simulink model "PVWIND"  (R2018a)
settings: Solver=FixedStepAuto  StartTime=0.0  StopTime=8  FixedStep=1e-4  RelTol=1e-3  EnableMultiTasking=on
InitFcn:
  | %clear all ;
  | %clc;
  | 
  | %%Wind System%%
  | 
  | %wind speed
  | Z_data=10;
  | Z_hub=85;
  | Z_0=0.03;
  | 
  | %Turbine
  | R_=45;
  | G=100;
  | lambda_opt=7.07;
  | Rho=1.225;
  | J=254;
  | f=0.01;
  | 
  | %RL filter;
  | 
  | fs=10000;
  | fe=50;
  | Ws=2*pi*fe;
  | Pres=3e6;
  | L=0.75e-3;
  | R=0.075;
  | c=38e-3;
  | 
  | %Commande CCR;
  | 
  | Id_=0;
  | Vdc_=1200;
  | %Vq_=0;
  | tr=0.001;
  | kp=3*L/tr;
  | ki=3*R/tr;
  | 
  | %CCM Commande;
  | 
  | p=2;
  | Tr=0.02;
  | Lfs=121e-6;
  | Lfr=57.3e-6;
  | Lm=12.12e-3;
  | m=1;
  | Ls=Lfs+Lm;
  | Lr=Lfr+m*Lm;
  | sigma=1-(m*Lm)^2/(Ls*Lr);
  | Rr=3.82e-3;
  | Rs=2.97e-3;
  | kpr=3*sigma*Lr/Tr;
  | kir=3*Rr/Tr;
  | Qs_ref=0;
  | 
  | %%PV SYSTEM%%
  | 
  | % T_cellule;
  | NOCT=45;
  | 
  | %PV module;
  | Ki=5e-4;
  | q=1.6e-19;
  | K=1.38e-23;
  | n=1.3;
  | Eg0=1.12;
  | Rs=.1;
  | Rp=515;
  | Tn=298.15;
  | Gn=1000;
  | Voc=46.5;
  | Isc=9.68;
  | Ns=72;
  | 
  | % Boost converter;
  | dv=3.1;   %53.85;
  | di=0.16;  %0.2053;
  | F=10000;
  | T=1/F;
  | %Vs=398;
  | Vab=690;         %sqrt(3)*Vs;
  | Vdc=1200;       %2*sqrt(2)*Vab/sqrt(3);
  | Vpv=303.2;
  | a=1-Vpv/Vdc;
  | Pn=350*40;
  | r=Vdc*Vdc/Pn;
  | l=0.5*Vpv*a*T/di;              %80e-3;
  | C=0.5*Vdc*a*T/(dv*r);       % 10e-6;
  | 
  | 
  | %Control PWM
  | Vgq=690/sqrt(3);
  | Fs=5000;
  | Ig=2*Pn/(3*690/sqrt(3)*sqrt(2));
  | dIg=0.05*Ig;
  | L1=690/(6*sqrt(2)*Fs*dIg);
  | R1=0.01;
  | 
  | 
  | tr1=1e-5;
  | Tau=tr1/3;
  | ki1=R1/Tau/Vgq;
  | kp1=L1/Tau/Vgq;
undefined symbols (not defined in the file or in its folder): sigbuilder_block
libraries: simulink x10, powerlib_meascontrol x10
(part 1 of 2)
settings Model: Creator=PC  LastModifiedBy=yassine
settings DataIOCC: SaveFormat=Array
settings OptimizationCC: LifeSpan=inf
settings DebuggingCC: SFUnexpectedBacktrackingDiag=warning  SFNoUnconditionalDefaultTransitionDiag=warning
settings CodeAppCC: StateflowObjectComments=on
settings GRTTargetCC: TargetLangStandard=C89/C90 (ANSI)
settings ConfigComp: CovMetricSettings=dw  CovSaveCumulativeToWorkspaceVar=on  CovSaveSingleToWorkspaceVar=on  CovExternalEMLEnable=off

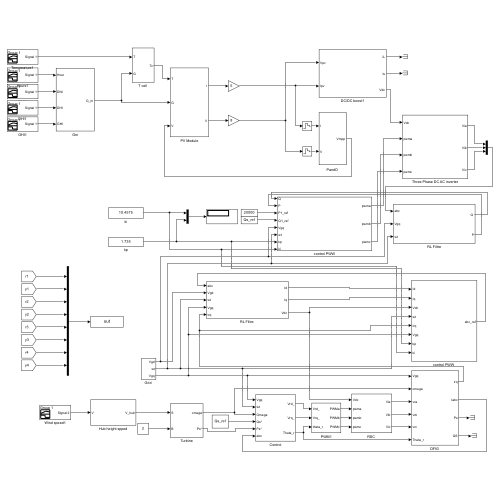
[thumbnail: Simulink's stored preview of the top-level diagram]
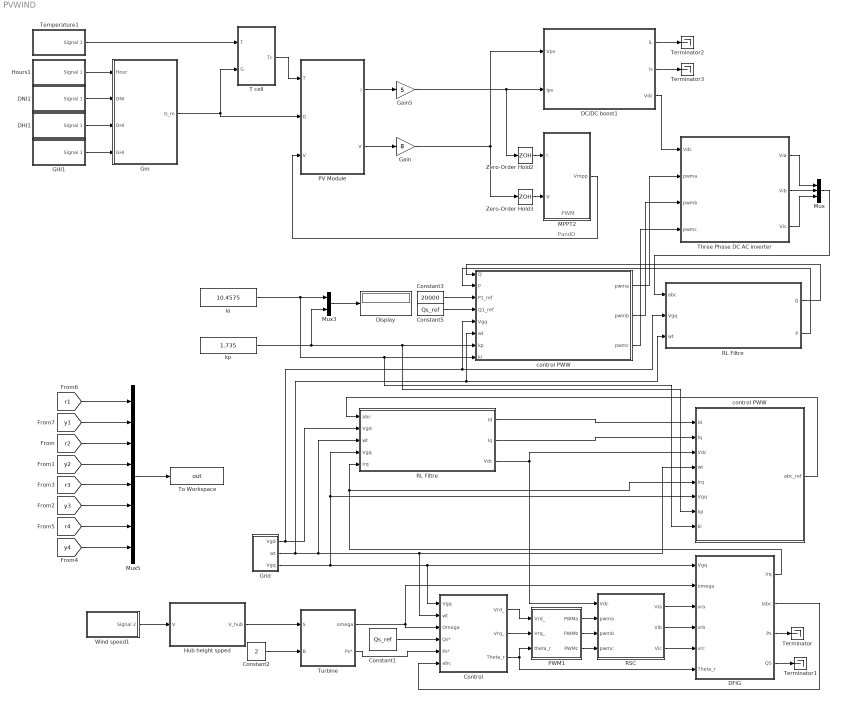
== system PVWIND ==
  note: PWM
  note: PandO
  Constant1 : Constant  Value=Qs_ref
  Constant2 : Constant  Value=2
  Constant3 : Constant  Value=20000
  Constant5 : Constant  Value=Qs_ref
  Control : Subsystem
  DC/DC boost1 : Subsystem
  "DFIG " : Subsystem
  DHI1 : Subsystem  Tag=STV Subsys  LoadFcn=sigbuilder_block('load');  StartFcn=sigbuilder_block('start');  StopFcn=sigbuilder_block('stop');  ClipboardFcn=sigbuilder_block('clipboard');  mask(Sigbuilder block){tuvar=[0:10]}
      mask help: Simulink:masks:SigbuilderBlock_MD
      mask init:
      | if ~strcmp(get_param(bdroot(gcbh),'SimulationStatus'),'stopped') tuvar = sigbuilder_block('maskInit'); end
      settings: CopyFcn=sigbuilder_block('copy');  DeleteFcn=sigbuilder_block('delete');  ModelCloseFcn=sigbuilder_block('modelClose');  PreSaveFcn=sigbuilder_block('preSave');  PauseFcn=sigbuilder_block('pause');  ContinueFcn=sigbuilder_block('continue');  NameChangeFcn=sigbuilder_block('namechange');  OpenFcn=sigbuilder_block('open',[303.6 90.6 550.8 400.2 ]);  CloseFcn=sigbuilder_block('close');
      mask Display: plot(0, 0, 100, 100,[2, 2, 32, 32, 2], [68, 8, 8, 68, 68],[32, 2], [38, 38], [32, 19, 2],[53, 60, 44], [32, 17, 17, 2],[16, 16, 31, 31]);txt = getActiveGroup(gcbh);text(2, 100, txt,'verticalAlignment', 'top');
  DNI1 : Subsystem  Tag=STV Subsys  LoadFcn=sigbuilder_block('load');  StartFcn=sigbuilder_block('start');  StopFcn=sigbuilder_block('stop');  ClipboardFcn=sigbuilder_block('clipboard');  mask(Sigbuilder block){tuvar=[0:10]}
      mask help: Simulink:masks:SigbuilderBlock_MD
      mask init:
      | if ~strcmp(get_param(bdroot(gcbh),'SimulationStatus'),'stopped') tuvar = sigbuilder_block('maskInit'); end
      settings: CopyFcn=sigbuilder_block('copy');  DeleteFcn=sigbuilder_block('delete');  ModelCloseFcn=sigbuilder_block('modelClose');  PreSaveFcn=sigbuilder_block('preSave');  PauseFcn=sigbuilder_block('pause');  ContinueFcn=sigbuilder_block('continue');  NameChangeFcn=sigbuilder_block('namechange');  OpenFcn=sigbuilder_block('open',[446.4 127.8 550.8 400.2 ]);  CloseFcn=sigbuilder_block('close');
      mask Display: plot(0, 0, 100, 100,[2, 2, 32, 32, 2], [68, 8, 8, 68, 68],[32, 2], [38, 38], [32, 19, 2],[53, 60, 44], [32, 17, 17, 2],[16, 16, 31, 31]);txt = getActiveGroup(gcbh);text(2, 100, txt,'verticalAlignment', 'top');
  Display : Display
  GHI1 : Subsystem  Tag=STV Subsys  LoadFcn=sigbuilder_block('load');  StartFcn=sigbuilder_block('start');  StopFcn=sigbuilder_block('stop');  ClipboardFcn=sigbuilder_block('clipboard');  mask(Sigbuilder block){tuvar=[0:10]}
      mask help: Simulink:masks:SigbuilderBlock_MD
      mask init:
      | if ~strcmp(get_param(bdroot(gcbh),'SimulationStatus'),'stopped') tuvar = sigbuilder_block('maskInit'); end
      settings: CopyFcn=sigbuilder_block('copy');  DeleteFcn=sigbuilder_block('delete');  ModelCloseFcn=sigbuilder_block('modelClose');  PreSaveFcn=sigbuilder_block('preSave');  PauseFcn=sigbuilder_block('pause');  ContinueFcn=sigbuilder_block('continue');  NameChangeFcn=sigbuilder_block('namechange');  OpenFcn=sigbuilder_block('open',[431.4 162.6 550.8 400.2 ]);  CloseFcn=sigbuilder_block('close');
      mask Display: plot(0, 0, 100, 100,[2, 2, 32, 32, 2], [68, 8, 8, 68, 68],[32, 2], [38, 38], [32, 19, 2],[53, 60, 44], [32, 17, 17, 2],[16, 16, 31, 31]);txt = getActiveGroup(gcbh);text(2, 100, txt,'verticalAlignment', 'top');
  Gain : Gain  Gain=8
  Gain5 : Gain  Gain=5
  Gm : Subsystem
  "Grid " : Subsystem
  Hours1 : Subsystem  Tag=STV Subsys  LoadFcn=sigbuilder_block('load');  StartFcn=sigbuilder_block('start');  StopFcn=sigbuilder_block('stop');  ClipboardFcn=sigbuilder_block('clipboard');  mask(Sigbuilder block){tuvar=[0:10]}
      mask help: Simulink:masks:SigbuilderBlock_MD
      mask init:
      | if ~strcmp(get_param(bdroot(gcbh),'SimulationStatus'),'stopped') tuvar = sigbuilder_block('maskInit'); end
      settings: CopyFcn=sigbuilder_block('copy');  DeleteFcn=sigbuilder_block('delete');  ModelCloseFcn=sigbuilder_block('modelClose');  PreSaveFcn=sigbuilder_block('preSave');  PauseFcn=sigbuilder_block('pause');  ContinueFcn=sigbuilder_block('continue');  NameChangeFcn=sigbuilder_block('namechange');  OpenFcn=sigbuilder_block('open',[446.4 139.2 550.8 400.2 ]);  CloseFcn=sigbuilder_block('close');
      mask Display: plot(0, 0, 100, 100,[2, 2, 32, 32, 2], [68, 8, 8, 68, 68],[32, 2], [38, 38], [32, 19, 2],[53, 60, 44], [32, 17, 17, 2],[16, 16, 31, 31]);txt = getActiveGroup(gcbh);text(2, 100, txt,'verticalAlignment', 'top');
  Hub height spped : Subsystem
  MPPT2 : Subsystem
  Mux : Mux  Inputs=3
  Mux3 : Mux  Inputs=2
  Mux5 : Mux  Inputs=8
  PV Module : Subsystem
  PWM1 : Subsystem
  RL Filtre : Subsystem
  "RL Filtre " : Subsystem
  "RSC " : Subsystem
  "T cell " : Subsystem
  Temperature1 : Subsystem  Tag=STV Subsys  LoadFcn=sigbuilder_block('load');  StartFcn=sigbuilder_block('start');  StopFcn=sigbuilder_block('stop');  ClipboardFcn=sigbuilder_block('clipboard');  mask(Sigbuilder block){tuvar=[0:10]}
      mask help: Simulink:masks:SigbuilderBlock_MD
      mask init:
      | if ~strcmp(get_param(bdroot(gcbh),'SimulationStatus'),'stopped') tuvar = sigbuilder_block('maskInit'); end
      settings: CopyFcn=sigbuilder_block('copy');  DeleteFcn=sigbuilder_block('delete');  ModelCloseFcn=sigbuilder_block('modelClose');  PreSaveFcn=sigbuilder_block('preSave');  PauseFcn=sigbuilder_block('pause');  ContinueFcn=sigbuilder_block('continue');  NameChangeFcn=sigbuilder_block('namechange');  OpenFcn=sigbuilder_block('open',[492.6 104.4 550.8 400.2 ]);  CloseFcn=sigbuilder_block('close');
      mask Display: plot(0, 0, 100, 100,[2, 2, 32, 32, 2], [68, 8, 8, 68, 68],[32, 2], [38, 38], [32, 19, 2],[53, 60, 44], [32, 17, 17, 2],[16, 16, 31, 31]);txt = getActiveGroup(gcbh);text(2, 100, txt,'verticalAlignment', 'top');
  Terminator{,1..3} (4 alike) : Terminator
  Three Phase DC AC inverter : Subsystem
  To Workspace : ToWorkspace  VariableName=out  SaveFormat=Timeseries  SampleTime=-1
  Turbine : Subsystem
  Wind speed1 : Subsystem  Tag=STV Subsys  LoadFcn=sigbuilder_block('load');  StartFcn=sigbuilder_block('start');  StopFcn=sigbuilder_block('stop');  ClipboardFcn=sigbuilder_block('clipboard');  mask(Sigbuilder block){tuvar=[0:10]}
      mask help: Simulink:masks:SigbuilderBlock_MD
      mask init:
      | if ~strcmp(get_param(bdroot(gcbh),'SimulationStatus'),'stopped') tuvar = sigbuilder_block('maskInit'); end
      settings: CopyFcn=sigbuilder_block('copy');  DeleteFcn=sigbuilder_block('delete');  ModelCloseFcn=sigbuilder_block('modelClose');  PreSaveFcn=sigbuilder_block('preSave');  PauseFcn=sigbuilder_block('pause');  ContinueFcn=sigbuilder_block('continue');  NameChangeFcn=sigbuilder_block('namechange');  OpenFcn=sigbuilder_block('open',[363 165 550.8 400.2 ]);  CloseFcn=sigbuilder_block('close');
      mask Display: plot(0, 0, 100, 100,[2, 2, 32, 32, 2], [68, 8, 8, 68, 68],[32, 2], [38, 38], [32, 19, 2],[53, 60, 44], [32, 17, 17, 2],[16, 16, 31, 31]);txt = getActiveGroup(gcbh);text(2, 100, txt,'verticalAlignment', 'top');
  Zero-Order Hold2 : ZeroOrderHold  SampleTime=1e-4
  Zero-Order Hold3 : ZeroOrderHold  SampleTime=1e-4
  control PWW : Subsystem
  "control PWW " : Subsystem
  ki : Constant  Value=10.4575
  kp : Constant  Value=1.735
  wires:
  "RSC "/1(Via) -> "DFIG "/3(vra)
  "RSC "/2(Vib) -> "DFIG "/4(vrb)
  "RSC "/3(Vic) -> "DFIG "/5(vrc)
  "RL Filtre "/3(Vdc) -> "RSC "/1(Vdc), "control PWW "/3(Vdc)
  PWM1/2(PWMb) -> "RSC "/3(pwmb)
  Control/1(Vrd_) -> PWM1/1(Vrd_)
  Control/2(Vrq_) -> PWM1/2(Vrq_)
  PWM1/1(PWMa) -> "RSC "/2(pwma)
  PWM1/3(PWMc) -> "RSC "/4(pwmc)
  "Grid "/3(Vgq) -> Control/1(Vgq), "DFIG "/1(Vgq), "RL Filtre "/4(Vgq), "control PWW "/6(Vgq)
  Control/3(Theta_r) -> "DFIG "/6(Theta_r), PWM1/3(theta_r)
  "DFIG "/2(Iabc) -> Control/6(abc)
  Turbine/1(omega) -> "DFIG "/2(omega), Control/3(Omega)
  "control PWW "/1(abc_ref) -> "RL Filtre "/1(abc)
  "RL Filtre "/1(Id) -> "control PWW "/1(Id)
  "RL Filtre "/2(Iq) -> "control PWW "/2(Iq)
  "DFIG "/1(irq) -> "RL Filtre "/5(Irq), "control PWW "/5(Irq)
  Constant1/1 -> Control/4(Qs*)
  Constant2/1 -> Turbine/2(B)
  Hub height spped/1(V_hub) -> Turbine/1(S)
  PV Module/2(V) -> Gain/1
  Zero-Order Hold2/1 -> MPPT2/1(I)
  Zero-Order Hold3/1 -> MPPT2/2(V)
  Gain/1 -> Zero-Order Hold3/1, DC/DC boost1/1(Vpv)
  "Grid "/1(Vgd) -> RL Filtre/2(Vgq), control PWW/5(Vgq), "RL Filtre "/2(Vgd)
  Constant5/1 -> control PWW/4(Q1_ref)
  Three Phase DC AC inverter/1(Via) -> Mux/1
  Three Phase DC AC inverter/2(Vib) -> Mux/2
  "Grid "/2(wt) -> Control/2(wt), "control PWW "/4(wt), "RL Filtre "/3(wt), RL Filtre/3(wt), control PWW/6(wt)
  Three Phase DC AC inverter/3(Vic) -> Mux/3
  DC/DC boost1/3(Vdc) -> Three Phase DC AC inverter/1(Vdc)
  MPPT2/1(Vmpp) -> PV Module/3("V ")
  PV Module/1(I) -> Gain5/1
  RL Filtre/1("Q ") -> control PWW/1("Q ")
  Mux/1 -> RL Filtre/1(abc)
  control PWW/1(pwma) -> Three Phase DC AC inverter/2(pwma)
  control PWW/2(pwmb) -> Three Phase DC AC inverter/3(pwmb)
  control PWW/3(pwmc) -> Three Phase DC AC inverter/4(pwmc)
  "T cell "/1(Tc) -> PV Module/1(T)
  Gain5/1 -> Zero-Order Hold2/1, DC/DC boost1/2(Ipv)
  Gm/1(G_m) -> "T cell "/2(G), PV Module/2(G)
  Hours1/1(Signal 1) -> Gm/1(Hour)
  DNI1/1(Signal 1) -> Gm/2(DNI)
  DHI1/1(Signal 1) -> Gm/3(DHI)
  GHI1/1(Signal 1) -> Gm/4(GHI)
  Temperature1/1(Signal 1) -> "T cell "/1(T)
  Wind speed1/1(Signal 2) -> Hub height spped/1(V)
  kp/1 -> "control PWW "/7(kp), control PWW/7(kp), Mux3/2
  ki/1 -> Mux3/1, "control PWW "/8(ki), control PWW/8(ki)
  Mux3/1 -> Display/1
  Constant3/1 -> control PWW/3(P1_ref)
  RL Filtre/2(P) -> control PWW/2(P)
  Turbine/2(Ps*) -> Control/5(Ps*)
  "DFIG "/3(Ps) -> Terminator/1
  "DFIG "/4(QS) -> Terminator1/1
  DC/DC boost1/1(iL) -> Terminator2/1
  DC/DC boost1/2(Is) -> Terminator3/1
  [r2] -> Mux5/3
  Mux5/1 -> To Workspace/1
  [y2] -> Mux5/4
  [r3] -> Mux5/5
  [y3] -> Mux5/6
  [r4] -> Mux5/7
  [y4] -> Mux5/8
  [y1] -> Mux5/2
  [r1] -> Mux5/1

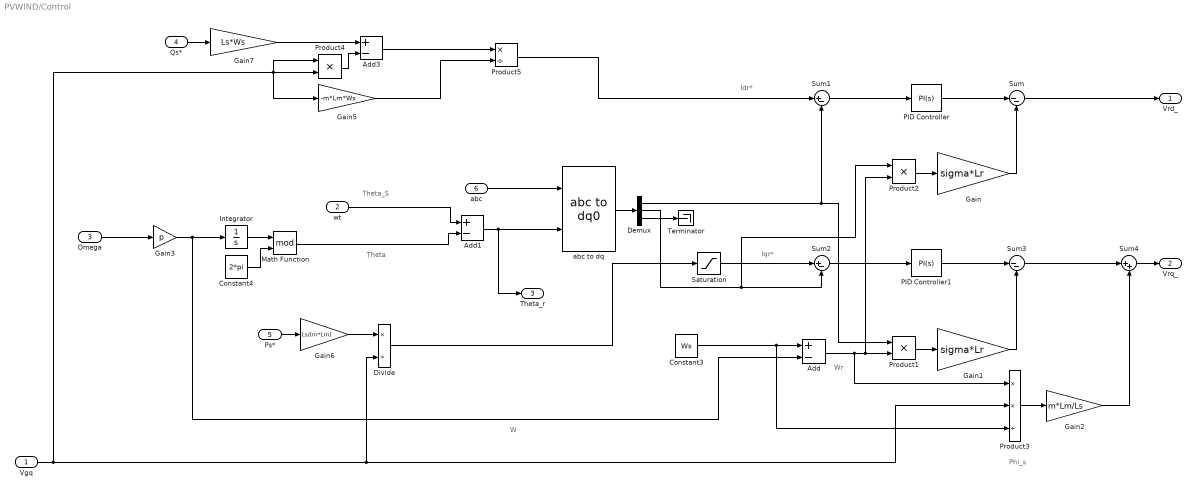
== system PVWIND/Control ==
  note: Theta_S
  note: Theta
  note: W
  note: Wr
  note: Phi_s
  note: Idr*
  note: Iqr*
  Vgq : Inport
  wt : Inport  Port=2
  Omega : Inport  Port=3
  Qs* : Inport  Port=4
  Ps* : Inport  Port=5
  abc : Inport  Port=6
  Add : Sum  Inputs=+-
  Add1 : Sum  Inputs=+-
  Add3 : Sum  Inputs=+-
  Constant3 : Constant  Value=Ws
  Constant4 : Constant  Value=2*pi
  Demux : Demux  Outputs=3
  Divide : Product  Inputs=*/
  Gain : Gain  Gain=sigma*Lr
  Gain1 : Gain  Gain=sigma*Lr
  Gain2 : Gain  Gain=m*Lm/Ls
  Gain3 : Gain  Gain=p
  Gain5 : Gain  Gain=-m*Lm*Ws
  Gain6 : Gain  Gain=Ls/(m*Lm)
  Gain7 : Gain  Gain=Ls*Ws
  Integrator : Integrator
  Math Function : Math  Operator=mod  SaturateOnIntegerOverflow=on
  PID Controller : simulink/Continuous/PID Controller  Controller=PI  Form=Parallel  TimeDomain=Continuous-time  SampleTime=-1  IntegratorMethod=Forward Euler  ControllerParametersSource=internal  P=kpr*62  I=kir*62  D=0  N=100  UseFilter=on  TunerSelectOption=Transfer Function Based (PID Tuner App)  InitialConditionSource=internal  InitialConditionForIntegrator=0  InitialConditionForFilter=0  DifferentiatorICPrevScaledInput=0  ExternalReset=none  TrackingMode=off  Kt=1  LimitOutput=off  UpperSaturationLimit=inf  LowerSaturationLimit=-inf  LinearizeAsGain=on  AntiWindupMode=none  Kb=1  POutMin=[]  POutMax=[]  IOutMin=[]  IOutMax=[]  DOutMin=[]  DOutMax=[]  NOutMin=[]  NOutMax=[]  SumOutMin=[]  SumOutMax=[]  SaturationOutMin=[]  SaturationOutMax=[]  PParamMin=[]  PParamMax=[]  IParamMin=[]  IParamMax=[]  DParamMin=[]  DParamMax=[]  NParamMin=[]  NParamMax=[]  KbParamMin=[]  KbParamMax=[]  KtParamMin=[]  KtParamMax=[]  KbOutMin=[]  KbOutMax=[]  KtOutMin=[]  KtOutMax=[]  IntegratorOutMin=[]  IntegratorOutMax=[]  FilterOutMin=[]  FilterOutMax=[]  SumI1OutMin=[]  SumI1OutMax=[]  SumI2OutMin=[]  SumI2OutMax=[]  SumI3OutMin=[]  SumI3OutMax=[]  SumDOutMin=[]  SumDOutMax=[]  DifferentiatorOutMin=[]  DifferentiatorOutMax=[]  FilterDiffOutCoefMin=[]  FilterDiffOutCoefMax=[]  ReciprocalOutMin=[]  ReciprocalOutMax=[]  SumDenOutMin=[]  SumDenOutMax=[]  SumNumOutMin=[]  SumNumOutMax=[]  DivideOutMin=[]  DivideOutMax=[]  IntegratorContinuousStateAttributes=''  IntegratorStateMustResolveToSignalObject=off  IntegratorRTWStateStorageClass=Auto  FilterContinuousStateAttributes=''  FilterStateMustResolveToSignalObject=off  FilterRTWStateStorageClass=Auto
  PID Controller1 : simulink/Continuous/PID Controller  Controller=PI  Form=Parallel  TimeDomain=Continuous-time  SampleTime=-1  IntegratorMethod=Forward Euler  ControllerParametersSource=internal  P=kpr*62  I=kir*62  D=0  N=100  UseFilter=on  TunerSelectOption=Transfer Function Based (PID Tuner App)  InitialConditionSource=internal  InitialConditionForIntegrator=0  InitialConditionForFilter=0  DifferentiatorICPrevScaledInput=0  ExternalReset=none  TrackingMode=off  Kt=1  LimitOutput=off  UpperSaturationLimit=inf  LowerSaturationLimit=-inf  LinearizeAsGain=on  AntiWindupMode=none  Kb=1  POutMin=[]  POutMax=[]  IOutMin=[]  IOutMax=[]  DOutMin=[]  DOutMax=[]  NOutMin=[]  NOutMax=[]  SumOutMin=[]  SumOutMax=[]  SaturationOutMin=[]  SaturationOutMax=[]  PParamMin=[]  PParamMax=[]  IParamMin=[]  IParamMax=[]  DParamMin=[]  DParamMax=[]  NParamMin=[]  NParamMax=[]  KbParamMin=[]  KbParamMax=[]  KtParamMin=[]  KtParamMax=[]  KbOutMin=[]  KbOutMax=[]  KtOutMin=[]  KtOutMax=[]  IntegratorOutMin=[]  IntegratorOutMax=[]  FilterOutMin=[]  FilterOutMax=[]  SumI1OutMin=[]  SumI1OutMax=[]  SumI2OutMin=[]  SumI2OutMax=[]  SumI3OutMin=[]  SumI3OutMax=[]  SumDOutMin=[]  SumDOutMax=[]  DifferentiatorOutMin=[]  DifferentiatorOutMax=[]  FilterDiffOutCoefMin=[]  FilterDiffOutCoefMax=[]  ReciprocalOutMin=[]  ReciprocalOutMax=[]  SumDenOutMin=[]  SumDenOutMax=[]  SumNumOutMin=[]  SumNumOutMax=[]  DivideOutMin=[]  DivideOutMax=[]  IntegratorContinuousStateAttributes=''  IntegratorStateMustResolveToSignalObject=off  IntegratorRTWStateStorageClass=Auto  FilterContinuousStateAttributes=''  FilterStateMustResolveToSignalObject=off  FilterRTWStateStorageClass=Auto
  Product1 : Product
  Product2 : Product
  Product3 : Product  Inputs=**/
  Product4 : Product  Inputs=**
  Product5 : Product  Inputs=*/
  Saturation : Saturate  UpperLimit=8e3  LowerLimit=-8e3
  Sum : Sum  Inputs=|--
  Sum1 : Sum  Inputs=|+-
  Sum2 : Sum  Inputs=|+-
  Sum3 : Sum  Inputs=|--
  Sum4 : Sum  Inputs=|++
  Terminator : Terminator
  abc to dq : powerlib_meascontrol/Transformations/abc to dq0  Alignment=90 degrees behind phase A axis
  Vrd_ : Outport
  Vrq_ : Outport  Port=2
  Theta_r : Outport  Port=3
  wires:
  Sum2/1 -> PID Controller1/1
  Sum1/1 -> PID Controller/1
  Demux/2 -> Sum2/2, Product2/1
  PID Controller/1 -> Sum/1
  Gain/1 -> Sum/2
  Sum4/1 -> Vrq_/1
  PID Controller1/1 -> Sum3/1
  Demux/1 -> Sum1/2, Product1/1
  Gain2/1 -> Sum4/2
  Sum3/1 -> Sum4/1
  Sum/1 -> Vrd_/1
  Gain1/1 -> Sum3/2
  Constant3/1 -> Product3/3, Add/1
  Product1/1 -> Gain1/1
  Add/1 -> Product3/1, Product2/2, Product1/2
  Omega/1 -> Gain3/1
  Product2/1 -> Gain/1
  Product3/1 -> Gain2/1
  abc to dq/1 -> Demux/1
  Demux/3 -> Terminator/1
  abc/1 -> abc to dq/1
  wt/1 -> Add1/1
  Integrator/1 -> Math Function/1
  Constant4/1 -> Math Function/2
  Math Function/1 -> Add1/2
  Gain3/1 -> Integrator/1, Add/2
  Add1/1 -> abc to dq/2, Theta_r/1
  Add3/1 -> Product5/1
  Vgq/1 -> Product3/2, Divide/2, Product4/1, Gain5/1, Product4/2
  Qs*/1 -> Gain7/1
  Gain5/1 -> Product5/2
  Product5/1 -> Sum1/1
  Ps*/1 -> Gain6/1
  Gain6/1 -> Divide/1
  Gain7/1 -> Add3/1
  Product4/1 -> Add3/2
  Divide/1 -> Saturation/1
  Saturation/1 -> Sum2/1

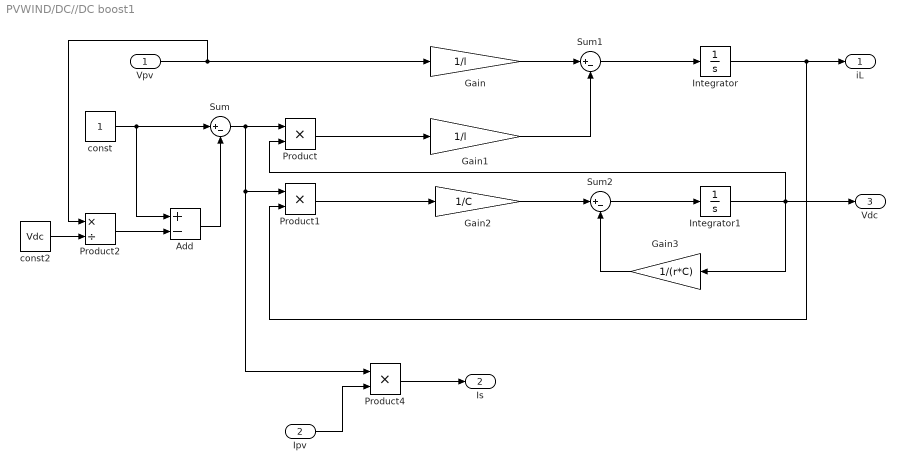
== system PVWIND/DC//DC boost1 ==
  Vpv : Inport
  Ipv : Inport  Port=2
  Add : Sum  Inputs=+-
  Gain : Gain  Gain=1/l
  Gain1 : Gain  Gain=1/l
  Gain2 : Gain  Gain=1/C
  Gain3 : Gain  Gain=1/(r*C)
  Integrator : Integrator
  Integrator1 : Integrator
  Product : Product
  Product1 : Product
  Product2 : Product  Inputs=*/
  Product4 : Product
  Sum : Sum  Inputs=|+-
  Sum1 : Sum  Inputs=|+-
  Sum2 : Sum  Inputs=|+-
  const : Constant
  const2 : Constant  Value=Vdc
  iL : Outport
  Is : Outport  Port=2
  Vdc : Outport  Port=3
  wires:
  Gain3/1 -> Sum2/2
  Integrator1/1 -> Vdc/1, Product/2, Gain3/1
  Sum2/1 -> Integrator1/1
  Product1/1 -> Gain2/1
  Product/1 -> Gain1/1
  Sum1/1 -> Integrator/1
  Gain1/1 -> Sum1/2
  Gain2/1 -> Sum2/1
  Gain/1 -> Sum1/1
  Add/1 -> Sum/2
  const/1 -> Add/1, Sum/1
  Vpv/1 -> Product2/1, Gain/1
  const2/1 -> Product2/2
  Product2/1 -> Add/2
  Sum/1 -> Product/1, Product4/1, Product1/1
  Integrator/1 -> iL/1, Product1/2
  Product4/1 -> Is/1
  Ipv/1 -> Product4/2

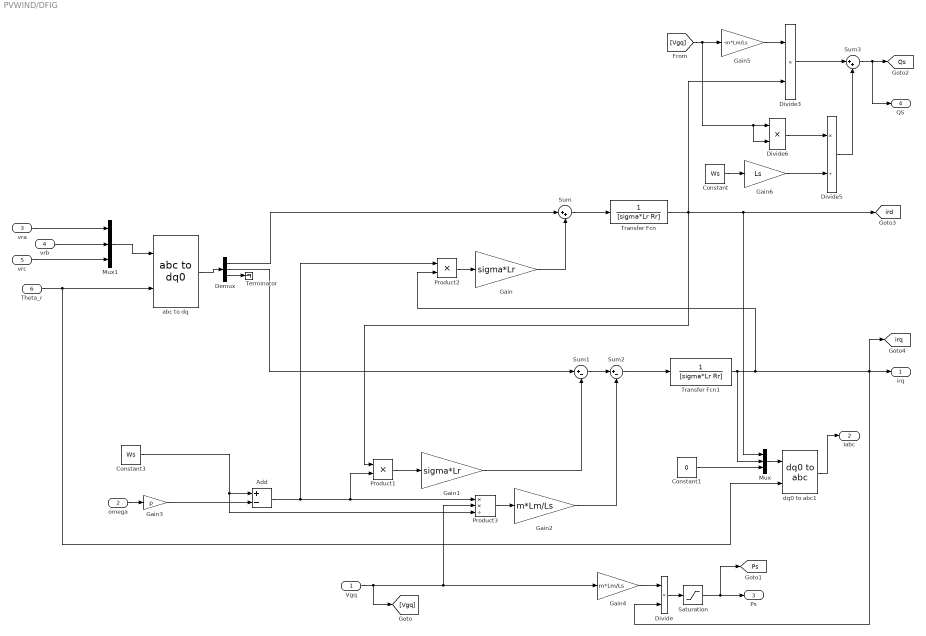
== system PVWIND/DFIG  ==
  Vgq : Inport
  omega : Inport  Port=2
  vra : Inport  Port=3
  vrb : Inport  Port=4
  vrc : Inport  Port=5
  Theta_r : Inport  Port=6
  Add : Sum  Inputs=+-
  Constant : Constant  Value=Ws
  Constant1 : Constant  Value=0
  Constant3 : Constant  Value=Ws
  Demux : Demux  Outputs=3
  Divide : Product  Inputs=**
  Divide3 : Product  Inputs=**
  Divide5 : Product  Inputs=*/
  Divide6 : Product  Inputs=**
  Gain : Gain  Gain=sigma*Lr
  Gain1 : Gain  Gain=sigma*Lr
  Gain2 : Gain  Gain=m*Lm/Ls
  Gain3 : Gain  Gain=p
  Gain4 : Gain  Gain=m*Lm/Ls
  Gain5 : Gain  Gain=-m*Lm/Ls
  Gain6 : Gain  Gain=Ls
  Mux : Mux  Inputs=3
  Mux1 : Mux  Inputs=3
  Product1 : Product
  Product2 : Product
  Product3 : Product  Inputs=**/
  Saturation : Saturate  UpperLimit=0  LowerLimit=-30e6
  Sum : Sum  Inputs=|++
  Sum1 : Sum  Inputs=|+-
  Sum2 : Sum  Inputs=|+-
  Sum3 : Sum  Inputs=|++
  Terminator : Terminator
  Transfer Fcn : TransferFcn  Denominator=[sigma*Lr Rr]
  Transfer Fcn1 : TransferFcn  Denominator=[sigma*Lr Rr]
  abc to dq : powerlib_meascontrol/Transformations/abc to dq0  Alignment=90 degrees behind phase A axis
  dq0 to abc1 : powerlib_meascontrol/Transformations/dq0 to abc  Alignment=90 degrees behind phase A axis
  irq : Outport
  Iabc : Outport  Port=2
  Ps : Outport  Port=3
  QS : Outport  Port=4
  tag scope: Ps=global, Qs=global, ird=global, irq=global
  wires:
  Transfer Fcn/1 -> [ird], Mux/1, Divide3/2, Product1/1
  Sum/1 -> Transfer Fcn/1
  Demux/2 -> Sum1/1
  Demux/1 -> Sum/1
  Product2/1 -> Gain/1
  Gain/1 -> Sum/2
  Constant3/1 -> Product3/3, Add/1
  Product1/1 -> Gain1/1
  Product3/1 -> Gain2/1
  Sum1/1 -> Sum2/1
  Gain1/1 -> Sum1/2
  Gain2/1 -> Sum2/2
  Sum2/1 -> Transfer Fcn1/1
  Add/1 -> Product2/1, Product1/2, Product3/1
  omega/1 -> Gain3/1
  Gain3/1 -> Add/2
  Constant1/1 -> Mux/3
  Mux/1 -> dq0 to abc1/1
  dq0 to abc1/1 -> Iabc/1
  abc to dq/1 -> Demux/1
  Demux/3 -> Terminator/1
  Mux1/1 -> abc to dq/1
  vra/1 -> Mux1/1
  vrb/1 -> Mux1/2
  vrc/1 -> Mux1/3
  Theta_r/1 -> dq0 to abc1/2, abc to dq/2
  Transfer Fcn1/1 -> [irq], irq/1, Divide/2, Product2/2, Mux/2
  Divide/1 -> Saturation/1
  Gain4/1 -> Divide/1
  Gain5/1 -> Divide3/1
  Divide3/1 -> Sum3/1
  Sum3/1 -> QS/1, [Qs]
  [Vgq] -> Divide6/2, Divide6/1, Gain5/1
  Divide6/1 -> Divide5/1
  Gain6/1 -> Divide5/2
  Constant/1 -> Gain6/1
  Divide5/1 -> Sum3/2
  Vgq/1 -> [Vgq], Product3/2, Gain4/1
  Saturation/1 -> Ps/1, [Ps]

== system PVWIND/DHI1 ==
  Demux : Demux  Tag=STV Demux  Outputs=1
      settings: DisplayOption=none
  FromWs : FromWorkspace  Tag=STV FromWs  VariableName=tuvar
      SigBuilderData=|
      | common.afterFinalStr = 'Extrapolate'
      | common.sampleTime = 0
      | dataSet.timeRange = [0 750]
      | dataSet.name = 'Group 1'
      | sbobj.Groups.Name = 'Group 1'
      | sbobj.Groups.Signals.Name = 'Signal 1'
      | sbobj.Groups.Signals.XData = [0 2 3 4 5 6 7 8 9 10 11 12 ... (744 elements, 1x744)]
      | sbobj.Groups.Signals.YData = [0 0 0 0 0 0 6 95 79 102 130 160 ... (744 elements, 1x744)]
      | sbobj.Groups.TimeRange = [0 750]
  Signal 1 : Outport  Tag=STV Outport
  wires:
  FromWs/1 -> Demux/1
  Demux/1 -> Signal 1/1

== system PVWIND/DNI1 ==
  Demux : Demux  Tag=STV Demux  Outputs=1
      settings: DisplayOption=none
  FromWs : FromWorkspace  Tag=STV FromWs  VariableName=tuvar
      SigBuilderData=|
      | common.afterFinalStr = 'Extrapolate'
      | common.sampleTime = 0
      | dataSet.timeRange = [0 750]
      | dataSet.name = 'Group 1'
      | sbobj.Groups.Name = 'Group 1'
      | sbobj.Groups.Signals.Name = 'Signal 1'
      | sbobj.Groups.Signals.XData = [0 2 3 4 5 6 7 8 9 10 11 12 ... (744 elements, 1x744)]
      | sbobj.Groups.Signals.YData = [0 0 0 0 0 0 0 325 691 784 826 833 ... (744 elements, 1x744)]
      | sbobj.Groups.TimeRange = [0 750]
  Signal 1 : Outport  Tag=STV Outport
  wires:
  FromWs/1 -> Demux/1
  Demux/1 -> Signal 1/1

== system PVWIND/GHI1 ==
  Demux : Demux  Tag=STV Demux  Outputs=1
      settings: DisplayOption=none
  FromWs : FromWorkspace  Tag=STV FromWs  VariableName=tuvar
      SigBuilderData=|
      | common.afterFinalStr = 'Extrapolate'
      | common.sampleTime = 0
      | dataSet.timeRange = [0 750]
      | dataSet.name = 'Group 1'
      | sbobj.Groups.Name = 'Group 1'
      | sbobj.Groups.Signals.Name = 'Signal 1'
      | sbobj.Groups.Signals.XData = [0 2 3 4 5 6 7 8 9 10 11 12 ... (744 elements, 1x744)]
      | sbobj.Groups.Signals.YData = [0 0 0 0 0 0 6 171 389 604 790 921 ... (744 elements, 1x744)]
      | sbobj.Groups.TimeRange = [0 750]
  Signal 1 : Outport  Tag=STV Outport
  wires:
  Demux/1 -> Signal 1/1
  FromWs/1 -> Demux/1

== system PVWIND/Gm ==
  Hour : Inport
  DNI : Inport  Port=2
  DHI : Inport  Port=3
  GHI : Inport  Port=4
  Irradiation : MATLAB Function  TreatAsAtomicUnit=on
  G_m : Outport
  wires:
  DHI/1 -> Irradiation/3(o)
  Irradiation/1(y) -> G_m/1
  DNI/1 -> Irradiation/2(k)
  GHI/1 -> Irradiation/4(p)
  Hour/1 -> Irradiation/1(i)

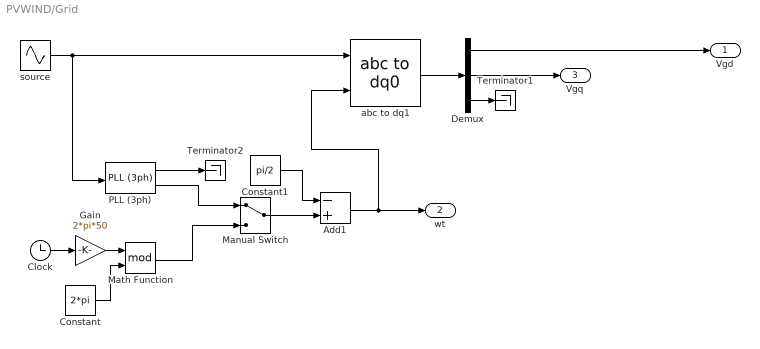
== system PVWIND/Grid  ==
  Add1 : Sum  Inputs=-+
  Clock : Clock
  Constant : Constant  Value=2*pi
  Constant1 : Constant  Value=pi/2
  Demux : Demux  Outputs=3
  Gain : Gain  Gain=2*pi*50
  Manual Switch : ManualSwitch
  Math Function : Math  Operator=mod  SaturateOnIntegerOverflow=on
  PLL (3ph) : powerlib_meascontrol/PLL/PLL (3ph)  Fmin=45  Par_Init=[0, 50]  ParK=[180, 3200, 1]  TcD=1e-4  MaxRateChangeFreq=12  FilterCutOffFreq=25  Ts=0  AGC=on
  Terminator1 : Terminator
  Terminator2 : Terminator
  abc to dq1 : powerlib_meascontrol/Transformations/abc to dq0  Alignment=90 degrees behind phase A axis
  source : Sin  Amplitude=690*sqrt(2)/sqrt(3)  Frequency=2*pi*50  Phase=[0 -2*pi/3 2*pi/3]  SampleTime=0
  Vgd : Outport
  wt : Outport  Port=2
  Vgq : Outport  Port=3
  wires:
  abc to dq1/1 -> Demux/1
  source/1 -> abc to dq1/1, PLL (3ph)/1
  Demux/2 -> Vgq/1
  Demux/3 -> Terminator1/1
  PLL (3ph)/1 -> Terminator2/1
  Clock/1 -> Gain/1
  PLL (3ph)/2 -> Manual Switch/1
  Gain/1 -> Math Function/1
  Constant/1 -> Math Function/2
  Math Function/1 -> Manual Switch/2
  Add1/1 -> abc to dq1/2, wt/1
  Constant1/1 -> Add1/1
  Manual Switch/1 -> Add1/2
  Demux/1 -> Vgd/1

== system PVWIND/Hours1 ==
  Demux : Demux  Tag=STV Demux  Outputs=1
      settings: DisplayOption=none
  FromWs : FromWorkspace  Tag=STV FromWs  VariableName=tuvar
      SigBuilderData=|
      | common.afterFinalStr = 'Extrapolate'
      | common.sampleTime = 0
      | dataSet.timeRange = [0 750]
      | dataSet.name = 'Group 1'
      | sbobj.Groups.Name = 'Group 1'
      | sbobj.Groups.Signals.Name = 'Signal 1'
      | sbobj.Groups.Signals.XData = [0 2 3 4 5 6 7 8 9 10 11 12 ... (746 elements, 1x746)]
      | sbobj.Groups.Signals.YData = [2 2 3 4 5 6 7 8 9 10 11 12 ... (746 elements, 1x746)]
      | sbobj.Groups.TimeRange = [0 750]
  Signal 1 : Outport  Tag=STV Outport
  wires:
  Demux/1 -> Signal 1/1
  FromWs/1 -> Demux/1

== system PVWIND/Hub height spped ==
  V : Inport
  Constant : Constant  Value=Z_hub
  Constant5 : Constant  Value=Z_data
  Constant6 : Constant  Value=Z_0
  Divide : Product  Inputs=*/
  Divide1 : Product  Inputs=*/
  Divide2 : Product  Inputs=*/
  Math Function : Math  Operator=log  SaturateOnIntegerOverflow=on
  Math Function1 : Math  Operator=log  SaturateOnIntegerOverflow=on
  Product : Product
  V_hub : Outport
  wires:
  Divide1/1 -> Math Function/1
  Divide2/1 -> Product/1
  Constant6/1 -> Divide1/2, Divide/2
  Constant5/1 -> Divide1/1
  Divide/1 -> Math Function1/1
  Constant/1 -> Divide/1
  Math Function1/1 -> Divide2/1
  Math Function/1 -> Divide2/2
  Product/1 -> V_hub/1
  V/1 -> Product/2

== system PVWIND/MPPT2 ==
  I : Inport
  V : Inport  Port=2
  CI : MATLAB Function  TreatAsAtomicUnit=on
  DP : Sum  Inputs=+-
  DV1 : Sum  Inputs=+-
  Memory2 : Memory
  Pk : Product  Inputs=**
  Pk-1 : Memory  InitialCondition=-0.1
  Unit Delay1 : UnitDelay  SampleTime=1e-4  HasFrameUpgradeWarning=on
  Vmpp : Outport
  wires:
  DP/1 -> CI/2(DP)
  DV1/1 -> CI/1(DV)
  CI/1(d) -> Unit Delay1/1
  Pk-1/1 -> DP/2
  Pk/1 -> Pk-1/1, DP/1
  V/1 -> Pk/1, Memory2/1, DV1/1
  Memory2/1 -> DV1/2
  I/1 -> Pk/2
  Unit Delay1/1 -> Vmpp/1

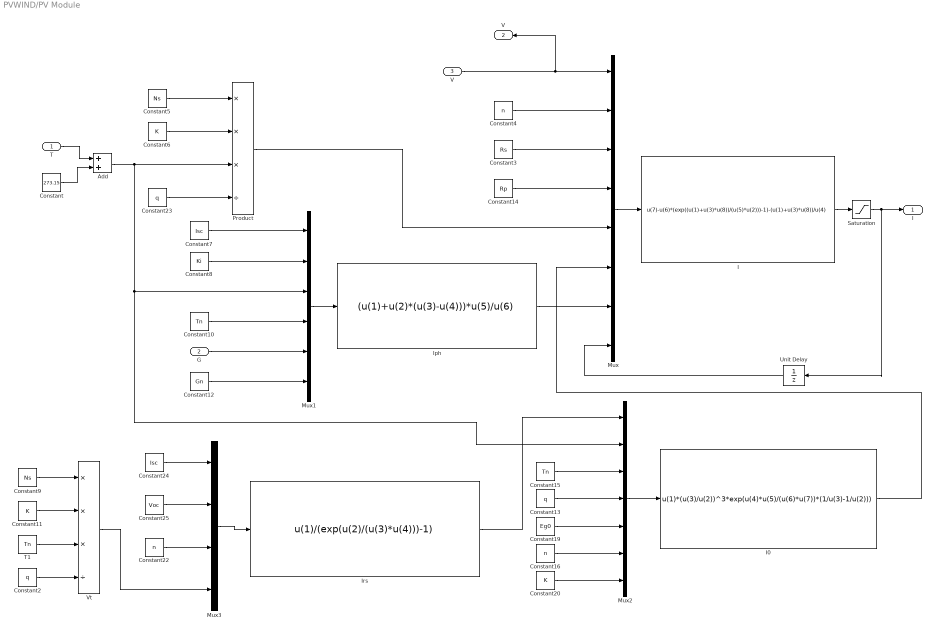
== system PVWIND/PV Module ==
  T : Inport
  G : Inport  Port=2
  "V " : Inport  Port=3
  Add : Sum
  Constant : Constant  Value=273.15
  Constant10 : Constant  Value=Tn
  Constant11 : Constant  Value=K
  Constant12 : Constant  Value=Gn
  Constant13 : Constant  Value=q
  Constant14 : Constant  Value=Rp
  Constant15 : Constant  Value=Tn
  Constant16 : Constant  Value=n
  Constant19 : Constant  Value=Eg0
  Constant2 : Constant  Value=q
  Constant20 : Constant  Value=K
  Constant22 : Constant  Value=n
  Constant23 : Constant  Value=q
  Constant24 : Constant  Value=Isc
  Constant25 : Constant  Value=Voc
  Constant3 : Constant  Value=Rs
  Constant4 : Constant  Value=n
  Constant5 : Constant  Value=Ns
  Constant6 : Constant  Value=K
  Constant7 : Constant  Value=Isc
  Constant8 : Constant  Value=Ki
  Constant9 : Constant  Value=Ns
  "I " : Fcn  Expr=u(7)-u(6)*(exp((u(1)+u(3)*u(8))/(u(5)*u(2)))-1)-(u(1)+u(3)*u(8))/u(4)
  I0 : Fcn  Expr=u(1)*(u(3)/u(2))^3*exp(u(4)*u(5)/(u(6)*u(7))*(1/u(3)-1/u(2)))
  Iph : Fcn  Expr=(u(1)+u(2)*(u(3)-u(4)))*u(5)/u(6)
  Irs : Fcn  Expr=u(1)/(exp(u(2)/(u(3)*u(4)))-1)
  Mux : Mux  Inputs=8
  Mux1 : Mux  Inputs=6
  Mux2 : Mux  Inputs=7
  Mux3 : Mux
  Product : Product  Inputs=***/
  Saturation : Saturate  UpperLimit=10  LowerLimit=0
  T1 : Constant  Value=Tn
  Unit Delay : UnitDelay  SampleTime=-1  HasFrameUpgradeWarning=on
  Vt : Product  Inputs=***/
  I : Outport
  V : Outport  Port=2
  wires:
  Constant5/1 -> Product/1
  Constant20/1 -> Mux2/7
  Constant4/1 -> Mux/2
  Constant3/1 -> Mux/3
  Product/1 -> Mux/5
  "V "/1 -> V/1, Mux/1
  Mux/1 -> "I "/1
  Constant14/1 -> Mux/4
  Mux1/1 -> Iph/1
  Constant8/1 -> Mux1/2
  Constant10/1 -> Mux1/4
  G/1 -> Mux1/5
  Iph/1 -> Mux/7
  Constant7/1 -> Mux1/1
  Constant12/1 -> Mux1/6
  Constant15/1 -> Mux2/3
  Mux2/1 -> I0/1
  Constant13/1 -> Mux2/4
  Constant19/1 -> Mux2/5
  I0/1 -> Mux/6
  Constant16/1 -> Mux2/6
  Add/1 -> Mux2/2, Mux1/3, Product/3
  Mux3/1 -> Irs/1
  Constant24/1 -> Mux3/1
  Constant22/1 -> Mux3/3
  Constant25/1 -> Mux3/2
  Irs/1 -> Mux2/1
  Constant2/1 -> Vt/4
  T1/1 -> Vt/3
  Constant9/1 -> Vt/1
  Constant11/1 -> Vt/2
  Vt/1 -> Mux3/4
  Constant6/1 -> Product/2
  Constant23/1 -> Product/4
  "I "/1 -> Saturation/1
  Constant/1 -> Add/2
  T/1 -> Add/1
  Saturation/1 -> I/1, Unit Delay/1
  Unit Delay/1 -> Mux/8

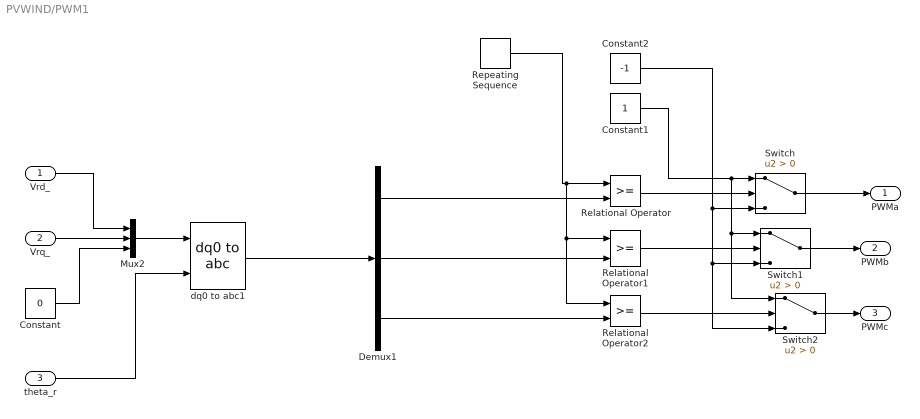
== system PVWIND/PWM1 ==
  Vrd_ : Inport
  Vrq_ : Inport  Port=2
  theta_r : Inport  Port=3
  Constant : Constant  Value=0
  Constant1 : Constant
  Constant2 : Constant  Value=-1
  Demux1 : Demux  Outputs=3
  Mux2 : Mux  Inputs=3
  Relational Operator : RelationalOperator  OutDataTypeStr=boolean  RndMeth=Nearest
  Relational Operator1 : RelationalOperator  OutDataTypeStr=boolean  RndMeth=Nearest
  Relational Operator2 : RelationalOperator  OutDataTypeStr=boolean  RndMeth=Nearest
  Repeating Sequence : simulink/Sources/Repeating Sequence  rep_seq_t=[0 1/40000 1/20000 3/40000 1/10000]  rep_seq_y="[0 600  0 -600 0]"
  Switch : Switch  Criteria=u2 > Threshold
  Switch1 : Switch  Criteria=u2 > Threshold
  Switch2 : Switch  Criteria=u2 > Threshold
  dq0 to abc1 : powerlib_meascontrol/Transformations/dq0 to abc  Alignment=90 degrees behind phase A axis
  PWMa : Outport
  PWMb : Outport  Port=2
  PWMc : Outport  Port=3
  wires:
  Constant/1 -> Mux2/3
  Switch2/1 -> PWMc/1
  Switch1/1 -> PWMb/1
  Switch/1 -> PWMa/1
  Demux1/2 -> Relational Operator1/2
  Demux1/3 -> Relational Operator2/2
  Demux1/1 -> Relational Operator/2
  Repeating Sequence/1 -> Relational Operator2/1, Relational Operator1/1, Relational Operator/1
  Constant2/1 -> Switch/3, Switch1/3, Switch2/3
  Mux2/1 -> dq0 to abc1/1
  Relational Operator2/1 -> Switch2/2
  Vrd_/1 -> Mux2/1
  Constant1/1 -> Switch1/1, Switch2/1, Switch/1
  Relational Operator/1 -> Switch/2
  Relational Operator1/1 -> Switch1/2
  Vrq_/1 -> Mux2/2
  theta_r/1 -> dq0 to abc1/2
  dq0 to abc1/1 -> Demux1/1

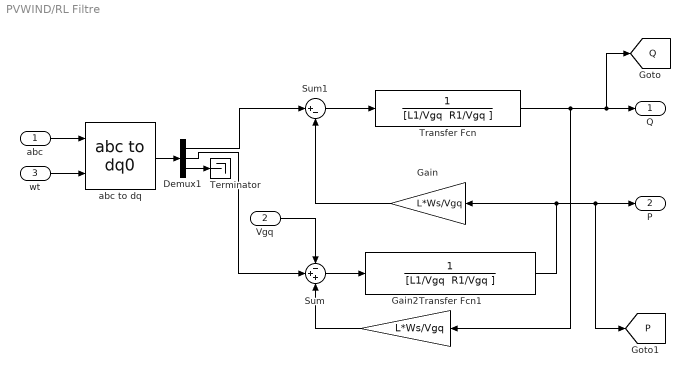
== system PVWIND/RL Filtre ==
  abc : Inport
  Vgq : Inport  Port=2
  wt : Inport  Port=3
  Demux1 : Demux  Outputs=3
  Gain : Gain  Gain=L*Ws/Vgq
  Gain2 : Gain  Gain=L*Ws/Vgq
  Sum : Sum  Inputs=-++
  Sum1 : Sum  Inputs=|+-
  Terminator : Terminator
  Transfer Fcn : TransferFcn  Denominator="[L1/Vgq  R1/Vgq ]"
  Transfer Fcn1 : TransferFcn  Denominator="[L1/Vgq  R1/Vgq ]"
  abc to dq : powerlib_meascontrol/Transformations/abc to dq0  Alignment=90 degrees behind phase A axis
  "Q " : Outport
  P : Outport  Port=2
  tag scope: P=global, Q=global
  wires:
  Transfer Fcn/1 -> [Q], "Q "/1, Gain2/1
  Demux1/1 -> Sum1/1
  Demux1/2 -> Sum/2
  abc to dq/1 -> Demux1/1
  Demux1/3 -> Terminator/1
  abc/1 -> abc to dq/1
  wt/1 -> abc to dq/2
  Vgq/1 -> Sum/1
  Gain2/1 -> Sum/3
  Gain/1 -> Sum1/2
  Sum1/1 -> Transfer Fcn/1
  Sum/1 -> Transfer Fcn1/1
  Transfer Fcn1/1 -> [P], P/1, Gain/1

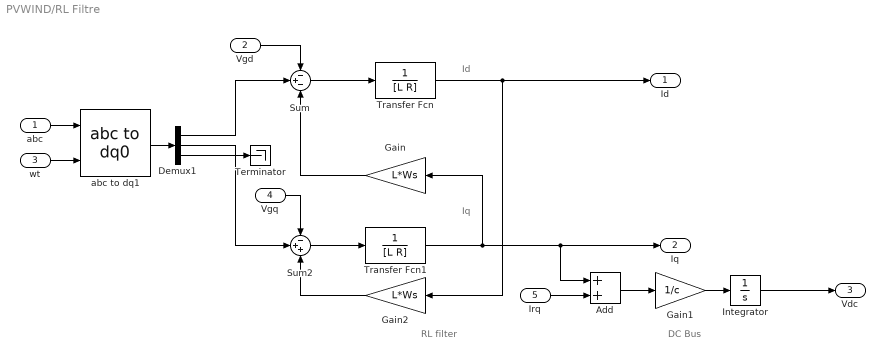
== system PVWIND/RL Filtre  ==
  note: RL filter
  note: DC Bus
  note: Id
  note: Iq
  abc : Inport
  Vgd : Inport  Port=2
  wt : Inport  Port=3
  Vgq : Inport  Port=4
  Irq : Inport  Port=5
  Add : Sum
  Demux1 : Demux  Outputs=3
  Gain : Gain  Gain=L*Ws
  Gain1 : Gain  Gain=1/c
  Gain2 : Gain  Gain=L*Ws
  Integrator : Integrator  UpperSaturationLimit=2000  LowerSaturationLimit=-2000
  Sum : Sum  Inputs=-+-
  Sum2 : Sum  Inputs=-++
  Terminator : Terminator
  Transfer Fcn : TransferFcn  Denominator=[L R]
  Transfer Fcn1 : TransferFcn  Denominator=[L R]
  abc to dq1 : powerlib_meascontrol/Transformations/abc to dq0  Alignment=90 degrees behind phase A axis
  Id : Outport
  Iq : Outport  Port=2
  Vdc : Outport  Port=3
  wires:
  Transfer Fcn1/1 -> Iq/1, Add/1, Gain/1
  abc to dq1/1 -> Demux1/1
  Demux1/3 -> Terminator/1
  abc/1 -> abc to dq1/1
  wt/1 -> abc to dq1/2
  Sum/1 -> Transfer Fcn/1
  Sum2/1 -> Transfer Fcn1/1
  Gain/1 -> Sum/3
  Gain2/1 -> Sum2/3
  Add/1 -> Gain1/1
  Gain1/1 -> Integrator/1
  Transfer Fcn/1 -> Id/1, Gain2/1
  Demux1/2 -> Sum2/2
  Demux1/1 -> Sum/2
  Irq/1 -> Add/2
  Vgq/1 -> Sum2/1
  Vgd/1 -> Sum/1
  Integrator/1 -> Vdc/1

== system PVWIND/RSC  ==
  Vdc : Inport
  pwma : Inport  Port=2
  pwmb : Inport  Port=3
  pwmc : Inport  Port=4
  Fcn : Fcn  Expr=u(1)/6*(2*u(2)-u(3)-u(4))
  Fcn1 : Fcn  Expr=u(1)/6*(-u(2)+2*u(3)-u(4))
  Fcn2 : Fcn  Expr=u(1)/6*(-u(2)-u(3)+2*u(4))
  Mux : Mux
  Via : Outport
  Vib : Outport  Port=2
  Vic : Outport  Port=3
  wires:
  Vdc/1 -> Mux/1
  Mux/1 -> Fcn2/1, Fcn1/1, Fcn/1
  pwma/1 -> Mux/2
  pwmb/1 -> Mux/3
  pwmc/1 -> Mux/4
  Fcn/1 -> Via/1
  Fcn1/1 -> Vib/1
  Fcn2/1 -> Vic/1

== system PVWIND/T cell  ==
  T : Inport
  G : Inport  Port=2
  Add : Sum  Inputs=+-
  Add1 : Sum
  Constant2 : Constant  Value=NOCT
  Constant4 : Constant  Value=20
  Gain1 : Gain  Gain=1/80
  Gain2 : Gain  Gain=1/10
  Product3 : Product
  Tc : Outport
  wires:
  Constant2/1 -> Add/1
  Product3/1 -> Gain1/1
  Constant4/1 -> Add/2
  Add/1 -> Product3/1
  Gain2/1 -> Product3/2
  Gain1/1 -> Add1/1
  G/1 -> Gain2/1
  T/1 -> Add1/2
  Add1/1 -> Tc/1

== system PVWIND/Temperature1 ==
  Demux : Demux  Tag=STV Demux  Outputs=1
      settings: DisplayOption=none
  FromWs : FromWorkspace  Tag=STV FromWs  VariableName=tuvar
      SigBuilderData=|
      | common.afterFinalStr = 'Extrapolate'
      | common.sampleTime = 0
      | dataSet.timeRange = [0 745]
      | dataSet.name = 'Group 1'
      | sbobj.Groups.Name = 'Group 1'
      | sbobj.Groups.Signals.Name = 'Signal 1'
      | sbobj.Groups.Signals.XData = [0 1 2 3 4 5 6 7 8 9 10 11 ... (746 elements, 1x746)]
      | sbobj.Groups.Signals.YData = [35.7 35.7 34 32.3 31.4 30.5 29.9 29.9 31.6 33.8 36 38.1 ... (746 elements, 1x746)]
      | sbobj.Groups.TimeRange = [0 745]
  Signal 1 : Outport  Tag=STV Outport
  wires:
  FromWs/1 -> Demux/1
  Demux/1 -> Signal 1/1

== system PVWIND/Three Phase DC AC inverter ==
  Vdc : Inport
  pwma : Inport  Port=2
  pwmb : Inport  Port=3
  pwmc : Inport  Port=4
  Fcn : Fcn  Expr=u(1)/6*(2*u(2)-u(3)-u(4))
  Fcn1 : Fcn  Expr=u(1)/6*(-u(2)+2*u(3)-u(4))
  Fcn2 : Fcn  Expr=u(1)/6*(-u(2)-u(3)+2*u(4))
  Mux : Mux
  Via : Outport
  Vib : Outport  Port=2
  Vic : Outport  Port=3
  wires:
  Vdc/1 -> Mux/1
  Mux/1 -> Fcn2/1, Fcn1/1, Fcn/1
  Fcn2/1 -> Vic/1
  Fcn1/1 -> Vib/1
  Fcn/1 -> Via/1
  pwma/1 -> Mux/2
  pwmb/1 -> Mux/3
  pwmc/1 -> Mux/4

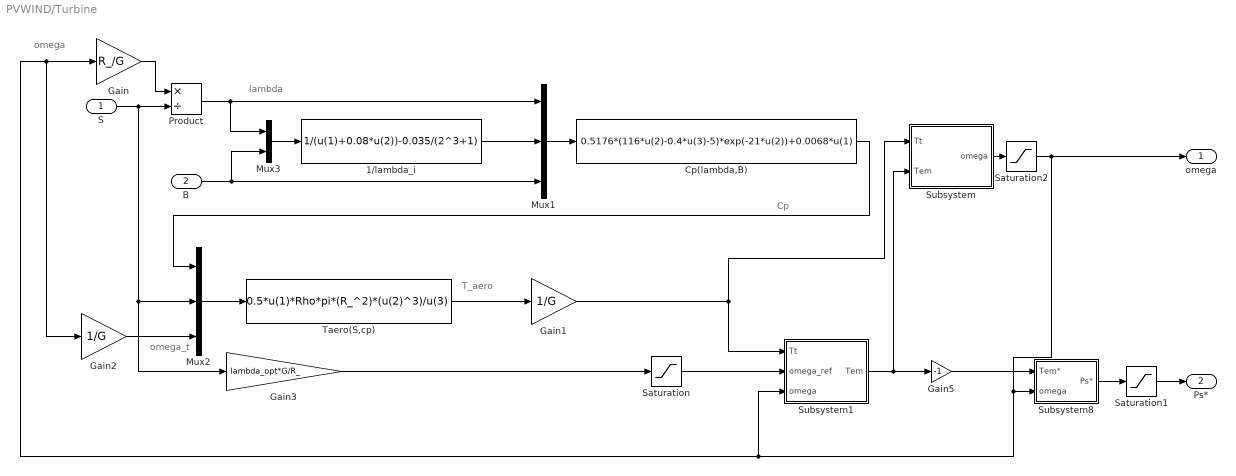
== system PVWIND/Turbine ==
  note: T_aero
  note: omega_t
  note: omega
  note: lambda
  note: Cp
  S : Inport
  B : Inport  Port=2
  1/lambda_i : Fcn  Expr=1/(u(1)+0.08*u(2))-0.035/(2^3+1)
  Cp(lambda,B) : Fcn  Expr=0.5176*(116*u(2)-0.4*u(3)-5)*exp(-21*u(2))+0.0068*u(1)
  Gain : Gain  Gain=R_/G
  Gain1 : Gain  Gain=1/G
  Gain2 : Gain  Gain=1/G
  Gain3 : Gain  Gain=lambda_opt*G/R_
  Gain5 : Gain  Gain=-1
  Mux1 : Mux  Inputs=3
  Mux2 : Mux  Inputs=3
  Mux3 : Mux  Inputs=2
  Product : Product  Inputs=*/
  Saturation : Saturate  UpperLimit=200  LowerLimit=0
  Saturation1 : Saturate  UpperLimit=0  LowerLimit=-3e6
  Saturation2 : Saturate  UpperLimit=200  LowerLimit=0
  Subsystem : Subsystem
  Subsystem1 : Subsystem
  Subsystem8 : Subsystem
  Taero(S,cp) : Fcn  Expr=0.5*u(1)*Rho*pi*(R_^2)*(u(2)^3)/u(3)
  omega : Outport
  Ps* : Outport  Port=2
  wires:
  Subsystem8/1(Ps*) -> Saturation1/1
  1/lambda_i/1 -> Mux1/2
  B/1 -> Mux1/3, Mux3/2
  Product/1 -> Mux3/1, Mux1/1
  S/1 -> Gain3/1, Mux2/2, Product/2
  Cp(lambda,B)/1 -> Mux2/1
  Gain/1 -> Product/1
  Gain2/1 -> Mux2/3
  Mux1/1 -> Cp(lambda,B)/1
  Mux2/1 -> Taero(S,cp)/1
  Taero(S,cp)/1 -> Gain1/1
  Mux3/1 -> 1/lambda_i/1
  Gain5/1 -> Subsystem8/1(Tem*)
  Subsystem1/1(Tem) -> Subsystem/2(Tem), Gain5/1
  Gain1/1 -> Subsystem1/1(Tt), Subsystem/1(Tt)
  Gain3/1 -> Saturation/1
  Saturation/1 -> Subsystem1/2(omega_ref)
  Saturation1/1 -> Ps*/1
  Subsystem/1(omega) -> Saturation2/1
  Saturation2/1 -> omega/1, Gain/1, Gain2/1, Subsystem1/3(omega), Subsystem8/2(omega)

== system PVWIND/Wind speed1 ==
  Demux : Demux  Tag=STV Demux  Outputs=1
      settings: DisplayOption=none
  FromWs : FromWorkspace  Tag=STV FromWs  VariableName=tuvar
      SigBuilderData=|
      | common.afterFinalStr = 'Extrapolate'
      | common.sampleTime = 0
      | dataSet.timeRange = [0 750]
      | dataSet.name = 'Group 1'
      | sbobj.Groups.Name = 'Group 1'
      | sbobj.Groups.Signals.Name = 'Signal 2'
      | sbobj.Groups.Signals.XData = [0 1 2 3 4 5 6 7 8 9 10 11 ... (745 elements, 1x745)]
      | sbobj.Groups.Signals.YData = [7.2 7.2 6.9 7.1 7.1 4.6 5.7 4.8 5.2 4.4 6.2 7.7 ... (745 elements, 1x745)]
      | sbobj.Groups.TimeRange = [0 750]
  Signal 2 : Outport  Tag=STV Outport
  wires:
  Demux/1 -> Signal 2/1
  FromWs/1 -> Demux/1

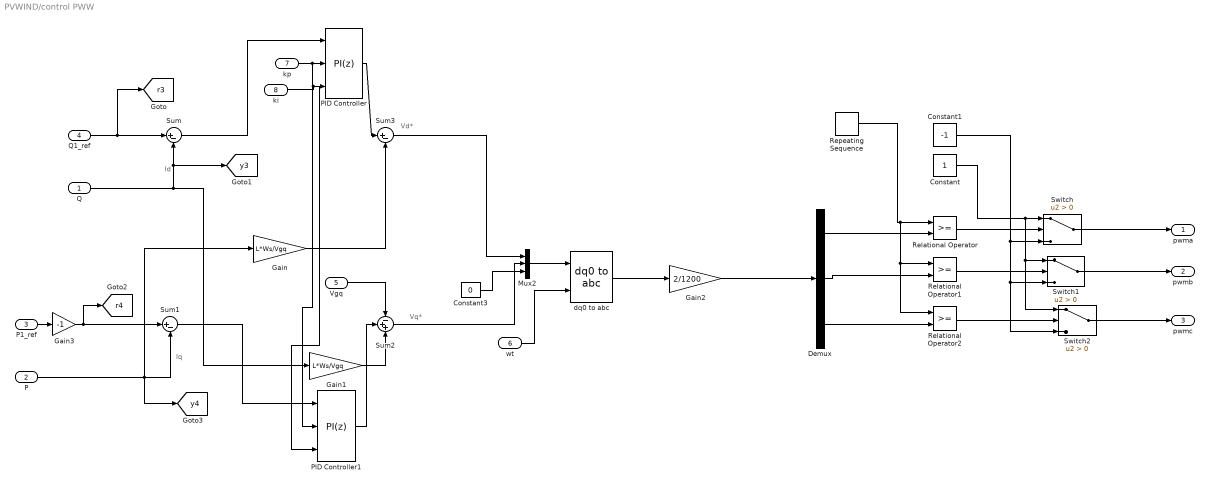
== system PVWIND/control PWW ==
  note: Vd*
  note: Vq*
  note: Iq
  note: Id
  "Q " : Inport
  P : Inport  Port=2
  P1_ref : Inport  Port=3
  Q1_ref : Inport  Port=4
  Vgq : Inport  Port=5
  wt : Inport  Port=6
  kp : Inport  Port=7
  ki : Inport  Port=8
  Constant : Constant
  Constant1 : Constant  Value=-1
  Constant3 : Constant  Value=0
  Demux : Demux  Outputs=3
  Gain : Gain  Gain=L*Ws/Vgq
  Gain1 : Gain  Gain=L*Ws/Vgq
  Gain2 : Gain  Gain=2/1200
  Gain3 : Gain  Gain=-1
  Mux2 : Mux  Inputs=3
  PID Controller : simulink/Continuous/PID Controller  Controller=PI  Form=Parallel  TimeDomain=Discrete-time  SampleTime=-1  IntegratorMethod=Forward Euler  ControllerParametersSource=external  P=1  I=1  D=0  N=100  UseFilter=off  TunerSelectOption=Transfer Function Based (PID Tuner App)  InitialConditionSource=internal  InitialConditionForIntegrator=0  InitialConditionForFilter=0  DifferentiatorICPrevScaledInput=0  ExternalReset=none  TrackingMode=off  Kt=1  LimitOutput=off  UpperSaturationLimit=inf  LowerSaturationLimit=-inf  LinearizeAsGain=on  AntiWindupMode=none  Kb=1  POutMin=[]  POutMax=[]  IOutMin=[]  IOutMax=[]  DOutMin=[]  DOutMax=[]  NOutMin=[]  NOutMax=[]  SumOutMin=[]  SumOutMax=[]  SaturationOutMin=[]  SaturationOutMax=[]  PParamMin=[]  PParamMax=[]  IParamMin=[]  IParamMax=[]  DParamMin=[]  DParamMax=[]  NParamMin=[]  NParamMax=[]  KbParamMin=[]  KbParamMax=[]  KtParamMin=[]  KtParamMax=[]  KbOutMin=[]  KbOutMax=[]  KtOutMin=[]  KtOutMax=[]  IntegratorOutMin=[]  IntegratorOutMax=[]  FilterOutMin=[]  FilterOutMax=[]  SumI1OutMin=[]  SumI1OutMax=[]  SumI2OutMin=[]  SumI2OutMax=[]  SumI3OutMin=[]  SumI3OutMax=[]  SumDOutMin=[]  SumDOutMax=[]  DifferentiatorOutMin=[]  DifferentiatorOutMax=[]  FilterDiffOutCoefMin=[]  FilterDiffOutCoefMax=[]  ReciprocalOutMin=[]  ReciprocalOutMax=[]  SumDenOutMin=[]  SumDenOutMax=[]  SumNumOutMin=[]  SumNumOutMax=[]  DivideOutMin=[]  DivideOutMax=[]  IntegratorContinuousStateAttributes=''  IntegratorStateMustResolveToSignalObject=off  IntegratorRTWStateStorageClass=Auto  FilterContinuousStateAttributes=''  FilterStateMustResolveToSignalObject=off  FilterRTWStateStorageClass=Auto
  PID Controller1 : simulink/Continuous/PID Controller  Controller=PI  Form=Parallel  TimeDomain=Discrete-time  SampleTime=-1  IntegratorMethod=Forward Euler  ControllerParametersSource=external  P=1  I=1  D=0  N=100  UseFilter=off  TunerSelectOption=Transfer Function Based (PID Tuner App)  InitialConditionSource=internal  InitialConditionForIntegrator=0  InitialConditionForFilter=0  DifferentiatorICPrevScaledInput=0  ExternalReset=none  TrackingMode=off  Kt=1  LimitOutput=off  UpperSaturationLimit=inf  LowerSaturationLimit=-inf  LinearizeAsGain=on  AntiWindupMode=none  Kb=1  POutMin=[]  POutMax=[]  IOutMin=[]  IOutMax=[]  DOutMin=[]  DOutMax=[]  NOutMin=[]  NOutMax=[]  SumOutMin=[]  SumOutMax=[]  SaturationOutMin=[]  SaturationOutMax=[]  PParamMin=[]  PParamMax=[]  IParamMin=[]  IParamMax=[]  DParamMin=[]  DParamMax=[]  NParamMin=[]  NParamMax=[]  KbParamMin=[]  KbParamMax=[]  KtParamMin=[]  KtParamMax=[]  KbOutMin=[]  KbOutMax=[]  KtOutMin=[]  KtOutMax=[]  IntegratorOutMin=[]  IntegratorOutMax=[]  FilterOutMin=[]  FilterOutMax=[]  SumI1OutMin=[]  SumI1OutMax=[]  SumI2OutMin=[]  SumI2OutMax=[]  SumI3OutMin=[]  SumI3OutMax=[]  SumDOutMin=[]  SumDOutMax=[]  DifferentiatorOutMin=[]  DifferentiatorOutMax=[]  FilterDiffOutCoefMin=[]  FilterDiffOutCoefMax=[]  ReciprocalOutMin=[]  ReciprocalOutMax=[]  SumDenOutMin=[]  SumDenOutMax=[]  SumNumOutMin=[]  SumNumOutMax=[]  DivideOutMin=[]  DivideOutMax=[]  IntegratorContinuousStateAttributes=''  IntegratorStateMustResolveToSignalObject=off  IntegratorRTWStateStorageClass=Auto  FilterContinuousStateAttributes=''  FilterStateMustResolveToSignalObject=off  FilterRTWStateStorageClass=Auto
  Relational Operator : RelationalOperator  OutDataTypeStr=boolean  RndMeth=Nearest
  Relational Operator1 : RelationalOperator  OutDataTypeStr=boolean  RndMeth=Nearest
  Relational Operator2 : RelationalOperator  OutDataTypeStr=boolean  RndMeth=Nearest
  Repeating Sequence : simulink/Sources/Repeating Sequence  rep_seq_t=[0 1/40000 1/20000 3/40000 1/10000]  rep_seq_y="[0 1  0 -1 0]"
  Sum : Sum  Inputs=|+-
  Sum1 : Sum  Inputs=|+-
  Sum2 : Sum  Inputs=-++
  Sum3 : Sum  Inputs=|+-
  Switch : Switch  Criteria=u2 > Threshold
  Switch1 : Switch  Criteria=u2 > Threshold
  Switch2 : Switch  Criteria=u2 > Threshold
  dq0 to abc : powerlib_meascontrol/Transformations/dq0 to abc  Alignment=90 degrees behind phase A axis
  pwma : Outport
  pwmb : Outport  Port=2
  pwmc : Outport  Port=3
  tag scope: r3=global, r4=global, y3=global, y4=global
  wires:
  Sum1/1 -> PID Controller1/1
  "Q "/1 -> Gain1/1, [y3], Sum/2
  Sum/1 -> PID Controller/1
  PID Controller/1 -> Sum3/1
  P1_ref/1 -> Gain3/1
  P/1 -> [y4], Gain/1, Sum1/2
  PID Controller1/1 -> Sum2/2
  Constant3/1 -> Mux2/3
  Q1_ref/1 -> [r3], Sum/1
  Repeating Sequence/1 -> Relational Operator2/1, Relational Operator1/1, Relational Operator/1
  Demux/1 -> Relational Operator/2
  Demux/2 -> Relational Operator1/2
  Demux/3 -> Relational Operator2/2
  Switch2/1 -> pwmc/1
  Switch1/1 -> pwmb/1
  Switch/1 -> pwma/1
  Relational Operator/1 -> Switch/2
  Constant/1 -> Switch1/1, Switch2/1, Switch/1
  Constant1/1 -> Switch/3, Switch1/3, Switch2/3
  Relational Operator1/1 -> Switch1/2
  Relational Operator2/1 -> Switch2/2
  Mux2/1 -> dq0 to abc/1
  Sum3/1 -> Mux2/1
  Sum2/1 -> Mux2/2
  wt/1 -> dq0 to abc/2
  Vgq/1 -> Sum2/1
  Gain/1 -> Sum3/2
  Gain1/1 -> Sum2/3
  dq0 to abc/1 -> Gain2/1
  Gain2/1 -> Demux/1
  Gain3/1 -> Sum1/1, [r4]
  kp/1 -> PID Controller1/2, PID Controller/2
  ki/1 -> PID Controller1/3, PID Controller/3

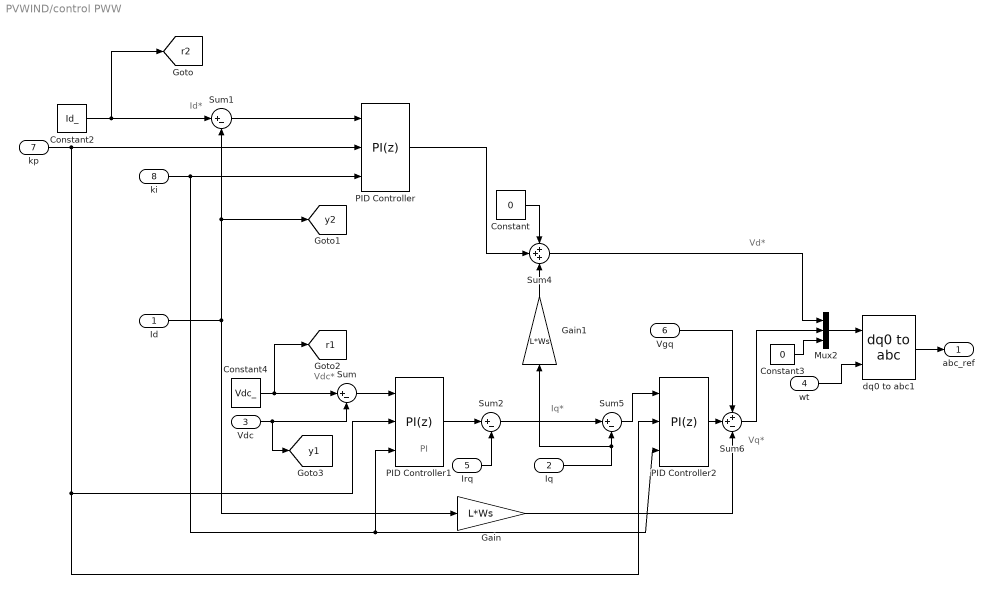
== system PVWIND/control PWW  ==
  note: Iq*
  note: Vq*
  note: Vd*
  note: Id*
  note: Vdc*
  note: PI
  Id : Inport
  Iq : Inport  Port=2
  Vdc : Inport  Port=3
  wt : Inport  Port=4
  Irq : Inport  Port=5
  Vgq : Inport  Port=6
  kp : Inport  Port=7
  ki : Inport  Port=8
  Constant : Constant  Value=0
  Constant2 : Constant  Value=Id_
  Constant3 : Constant  Value=0
  Constant4 : Constant  Value=Vdc_
  Gain : Gain  Gain=L*Ws
  Gain1 : Gain  Gain=L*Ws
  Mux2 : Mux  Inputs=3
  PID Controller : simulink/Continuous/PID Controller  Controller=PI  Form=Parallel  TimeDomain=Discrete-time  SampleTime=-1  IntegratorMethod=Forward Euler  ControllerParametersSource=external  P=1  I=1  D=0  N=100  UseFilter=off  TunerSelectOption=Transfer Function Based (PID Tuner App)  InitialConditionSource=internal  InitialConditionForIntegrator=0  InitialConditionForFilter=0  DifferentiatorICPrevScaledInput=0  ExternalReset=none  TrackingMode=off  Kt=1  LimitOutput=off  UpperSaturationLimit=inf  LowerSaturationLimit=-inf  LinearizeAsGain=on  AntiWindupMode=none  Kb=1  POutMin=[]  POutMax=[]  IOutMin=[]  IOutMax=[]  DOutMin=[]  DOutMax=[]  NOutMin=[]  NOutMax=[]  SumOutMin=[]  SumOutMax=[]  SaturationOutMin=[]  SaturationOutMax=[]  PParamMin=[]  PParamMax=[]  IParamMin=[]  IParamMax=[]  DParamMin=[]  DParamMax=[]  NParamMin=[]  NParamMax=[]  KbParamMin=[]  KbParamMax=[]  KtParamMin=[]  KtParamMax=[]  KbOutMin=[]  KbOutMax=[]  KtOutMin=[]  KtOutMax=[]  IntegratorOutMin=[]  IntegratorOutMax=[]  FilterOutMin=[]  FilterOutMax=[]  SumI1OutMin=[]  SumI1OutMax=[]  SumI2OutMin=[]  SumI2OutMax=[]  SumI3OutMin=[]  SumI3OutMax=[]  SumDOutMin=[]  SumDOutMax=[]  DifferentiatorOutMin=[]  DifferentiatorOutMax=[]  FilterDiffOutCoefMin=[]  FilterDiffOutCoefMax=[]  ReciprocalOutMin=[]  ReciprocalOutMax=[]  SumDenOutMin=[]  SumDenOutMax=[]  SumNumOutMin=[]  SumNumOutMax=[]  DivideOutMin=[]  DivideOutMax=[]  IntegratorContinuousStateAttributes=''  IntegratorStateMustResolveToSignalObject=off  IntegratorRTWStateStorageClass=Auto  FilterContinuousStateAttributes=''  FilterStateMustResolveToSignalObject=off  FilterRTWStateStorageClass=Auto
  PID Controller1 : simulink/Continuous/PID Controller  Controller=PI  Form=Parallel  TimeDomain=Discrete-time  SampleTime=-1  IntegratorMethod=Forward Euler  ControllerParametersSource=external  P=1  I=1  D=0  N=100  UseFilter=off  TunerSelectOption=Transfer Function Based (PID Tuner App)  InitialConditionSource=internal  InitialConditionForIntegrator=0  InitialConditionForFilter=0  DifferentiatorICPrevScaledInput=0  ExternalReset=none  TrackingMode=off  Kt=1  LimitOutput=off  UpperSaturationLimit=inf  LowerSaturationLimit=-inf  LinearizeAsGain=on  AntiWindupMode=none  Kb=1  POutMin=[]  POutMax=[]  IOutMin=[]  IOutMax=[]  DOutMin=[]  DOutMax=[]  NOutMin=[]  NOutMax=[]  SumOutMin=[]  SumOutMax=[]  SaturationOutMin=[]  SaturationOutMax=[]  PParamMin=[]  PParamMax=[]  IParamMin=[]  IParamMax=[]  DParamMin=[]  DParamMax=[]  NParamMin=[]  NParamMax=[]  KbParamMin=[]  KbParamMax=[]  KtParamMin=[]  KtParamMax=[]  KbOutMin=[]  KbOutMax=[]  KtOutMin=[]  KtOutMax=[]  IntegratorOutMin=[]  IntegratorOutMax=[]  FilterOutMin=[]  FilterOutMax=[]  SumI1OutMin=[]  SumI1OutMax=[]  SumI2OutMin=[]  SumI2OutMax=[]  SumI3OutMin=[]  SumI3OutMax=[]  SumDOutMin=[]  SumDOutMax=[]  DifferentiatorOutMin=[]  DifferentiatorOutMax=[]  FilterDiffOutCoefMin=[]  FilterDiffOutCoefMax=[]  ReciprocalOutMin=[]  ReciprocalOutMax=[]  SumDenOutMin=[]  SumDenOutMax=[]  SumNumOutMin=[]  SumNumOutMax=[]  DivideOutMin=[]  DivideOutMax=[]  IntegratorContinuousStateAttributes=''  IntegratorStateMustResolveToSignalObject=off  IntegratorRTWStateStorageClass=Auto  FilterContinuousStateAttributes=''  FilterStateMustResolveToSignalObject=off  FilterRTWStateStorageClass=Auto
  PID Controller2 : simulink/Continuous/PID Controller  Controller=PI  Form=Parallel  TimeDomain=Discrete-time  SampleTime=-1  IntegratorMethod=Forward Euler  ControllerParametersSource=external  P=1  I=1  D=0  N=100  UseFilter=off  TunerSelectOption=Transfer Function Based (PID Tuner App)  InitialConditionSource=internal  InitialConditionForIntegrator=0  InitialConditionForFilter=0  DifferentiatorICPrevScaledInput=0  ExternalReset=none  TrackingMode=off  Kt=1  LimitOutput=off  UpperSaturationLimit=inf  LowerSaturationLimit=-inf  LinearizeAsGain=on  AntiWindupMode=none  Kb=1  POutMin=[]  POutMax=[]  IOutMin=[]  IOutMax=[]  DOutMin=[]  DOutMax=[]  NOutMin=[]  NOutMax=[]  SumOutMin=[]  SumOutMax=[]  SaturationOutMin=[]  SaturationOutMax=[]  PParamMin=[]  PParamMax=[]  IParamMin=[]  IParamMax=[]  DParamMin=[]  DParamMax=[]  NParamMin=[]  NParamMax=[]  KbParamMin=[]  KbParamMax=[]  KtParamMin=[]  KtParamMax=[]  KbOutMin=[]  KbOutMax=[]  KtOutMin=[]  KtOutMax=[]  IntegratorOutMin=[]  IntegratorOutMax=[]  FilterOutMin=[]  FilterOutMax=[]  SumI1OutMin=[]  SumI1OutMax=[]  SumI2OutMin=[]  SumI2OutMax=[]  SumI3OutMin=[]  SumI3OutMax=[]  SumDOutMin=[]  SumDOutMax=[]  DifferentiatorOutMin=[]  DifferentiatorOutMax=[]  FilterDiffOutCoefMin=[]  FilterDiffOutCoefMax=[]  ReciprocalOutMin=[]  ReciprocalOutMax=[]  SumDenOutMin=[]  SumDenOutMax=[]  SumNumOutMin=[]  SumNumOutMax=[]  DivideOutMin=[]  DivideOutMax=[]  IntegratorContinuousStateAttributes=''  IntegratorStateMustResolveToSignalObject=off  IntegratorRTWStateStorageClass=Auto  FilterContinuousStateAttributes=''  FilterStateMustResolveToSignalObject=off  FilterRTWStateStorageClass=Auto
  Sum{,1..2,5} (4 alike) : Sum  Inputs=|+-
  Sum4 : Sum  Inputs=+++
  Sum6 : Sum  Inputs=++-
  dq0 to abc1 : powerlib_meascontrol/Transformations/dq0 to abc  Alignment=90 degrees behind phase A axis
  abc_ref : Outport
  tag scope: r1=global, r2=global, y1=global, y2=global
  wires:
  Sum1/1 -> PID Controller/1
  Sum/1 -> PID Controller1/1
  PID Controller1/1 -> Sum2/1
  PID Controller/1 -> Sum4/2
  Constant3/1 -> Mux2/3
  Mux2/1 -> dq0 to abc1/1
  dq0 to abc1/1 -> abc_ref/1
  wt/1 -> dq0 to abc1/2
  PID Controller2/1 -> Sum6/2
  Sum6/1 -> Mux2/2
  Sum5/1 -> PID Controller2/1
  Sum4/1 -> Mux2/1
  Vgq/1 -> Sum6/1
  Gain/1 -> Sum6/3
  Irq/1 -> Sum2/2
  Constant/1 -> Sum4/1
  Gain1/1 -> Sum4/3
  Sum2/1 -> Sum5/1
  Iq/1 -> Sum5/2, Gain1/1
  Constant4/1 -> Sum/1, [r1]
  Vdc/1 -> Sum/2, [y1]
  kp/1 -> PID Controller1/2, PID Controller2/2, PID Controller/2
  ki/1 -> PID Controller/3, PID Controller1/3, PID Controller2/3
  Id/1 -> Gain/1, [y2], Sum1/2
  Constant2/1 -> [r2], Sum1/1

== system PVWIND/Turbine/Subsystem ==
  Tt : Inport
  Tem : Inport  Port=2
  Add : Sum  Inputs=+--
  Gain6 : Gain  Gain=1/J
  Gain7 : Gain  Gain=f
  Integrator : Integrator  InitialCondition=64.5  LowerSaturationLimit=1e-5
  omega : Outport
  wires:
  Add/1 -> Gain6/1
  Integrator/1 -> omega/1, Gain7/1
  Gain6/1 -> Integrator/1
  Tt/1 -> Add/1
  Gain7/1 -> Add/3
  Tem/1 -> Add/2

== system PVWIND/Turbine/Subsystem1 ==
  Tt : Inport
  omega_ref : Inport  Port=2
  omega : Inport  Port=3
  Add : Sum  Inputs=+-
  PID Controller : simulink/Continuous/PID Controller  Controller=PI  Form=Parallel  TimeDomain=Continuous-time  SampleTime=-1  IntegratorMethod=Forward Euler  ControllerParametersSource=internal  P=J  I=f  D=0  N=100  UseFilter=on  TunerSelectOption=Transfer Function Based (PID Tuner App)  InitialConditionSource=internal  InitialConditionForIntegrator=0  InitialConditionForFilter=0  DifferentiatorICPrevScaledInput=0  ExternalReset=none  TrackingMode=off  Kt=1  LimitOutput=off  UpperSaturationLimit=inf  LowerSaturationLimit=0  LinearizeAsGain=on  AntiWindupMode=none  Kb=1  POutMin=[]  POutMax=[]  IOutMin=[]  IOutMax=[]  DOutMin=[]  DOutMax=[]  NOutMin=[]  NOutMax=[]  SumOutMin=[]  SumOutMax=[]  SaturationOutMin=[]  SaturationOutMax=[]  PParamMin=[]  PParamMax=[]  IParamMin=[]  IParamMax=[]  DParamMin=[]  DParamMax=[]  NParamMin=[]  NParamMax=[]  KbParamMin=[]  KbParamMax=[]  KtParamMin=[]  KtParamMax=[]  KbOutMin=[]  KbOutMax=[]  KtOutMin=[]  KtOutMax=[]  IntegratorOutMin=[]  IntegratorOutMax=[]  FilterOutMin=[]  FilterOutMax=[]  SumI1OutMin=[]  SumI1OutMax=[]  SumI2OutMin=[]  SumI2OutMax=[]  SumI3OutMin=[]  SumI3OutMax=[]  SumDOutMin=[]  SumDOutMax=[]  DifferentiatorOutMin=[]  DifferentiatorOutMax=[]  FilterDiffOutCoefMin=[]  FilterDiffOutCoefMax=[]  ReciprocalOutMin=[]  ReciprocalOutMax=[]  SumDenOutMin=[]  SumDenOutMax=[]  SumNumOutMin=[]  SumNumOutMax=[]  DivideOutMin=[]  DivideOutMax=[]  IntegratorContinuousStateAttributes=''  IntegratorStateMustResolveToSignalObject=off  IntegratorRTWStateStorageClass=Auto  FilterContinuousStateAttributes=''  FilterStateMustResolveToSignalObject=off  FilterRTWStateStorageClass=Auto
  Saturation : Saturate  UpperLimit=1.9e4  LowerLimit=0
  Sum3 : Sum  Inputs=|+-
  Tem : Outport
  wires:
  Tt/1 -> Add/1
  Saturation/1 -> Tem/1
  Add/1 -> Saturation/1
  PID Controller/1 -> Add/2
  omega_ref/1 -> Sum3/1
  Sum3/1 -> PID Controller/1
  omega/1 -> Sum3/2

== system PVWIND/Turbine/Subsystem8 ==
  Tem* : Inport
  omega : Inport  Port=2
  Gain : Gain
  Mux : Mux  Inputs=2
  fcn2 : Fcn  Expr=u(1)*u(2)
  Ps* : Outport
  wires:
  Gain/1 -> Mux/2
  Tem*/1 -> Mux/1
  fcn2/1 -> Ps*/1
  omega/1 -> Gain/1
  Mux/1 -> fcn2/1
